simulink model "DBX_control_harness"  (R2015a)
settings: Solver=ode2  SolverMode=SingleTasking  StartTime=0.0  StopTime=inf  FixedStep=T_sim  RelTol=1e-3
values from neighbouring files (symbols this model uses):
  airport_alt = 587.5    [Run_DBX.m]
  latitude = 40.463650    (= 40.46365)    [Run_DBX.m]
  longitude = -3.554389    [Run_DBX.m]
  T_ctrl = 0.01    [Run_DBX.m]
  T_sim = 0.01    [Run_DBX.m]
undefined symbols (not defined in the file or in its folder): accel_sigmas, Alt_0, DBX_PWM, delta_a_L_0_servo, delta_a_R_0_servo, delta_rv_L_0_servo, delta_rv_R_0_servo, eta_1_0_servo, eta_2_0_servo, eta_3_0_servo, Euler_0, Euler_dot_sigmas, Euler_sigmas, g, GPS_pos_sig, Initial_Omegas, Newton, omgea_b_sigmas, qbar_sigma, quaternion_sigmas, Raphson, Roll_pich_sens, sigbuilder_block, Speed_sigmas, TAS_0, tau_1_0, tau_2_0, tau_3_0, Throtle_sens, Volt_noise, Yaw_sens
libraries: DBX_model x14, commnoisgen2 x9, simulink x3, powerlib_meascontrol x2, utility x1
(part 2 of 2)

== system DBX_control_harness/DBX FCS/PWM Interface out/PWM Interface out: Agosto prototipo ==
  PWM1 : Inport
  PWM2 : Inport  Port=2
  PWM3 : Inport  Port=3
  PWM4 : Inport  Port=4
  PWM5 : Inport  Port=5
  PWM6 : Inport  Port=6
  PWM7 : Inport  Port=7
  PWM8 : Inport  Port=8
  Constant : Constant  Value=1500
  Constant1 : Constant  Value=1100
  Mux : Mux  Inputs=3
  Mux1 : Mux  Inputs=7
  Motores : Outport
  Servos : Outport  Port=2
  wires:
  Mux/1 -> Motores/1
  Mux1/1 -> Servos/1
  PWM1/1 -> Mux/1
  PWM2/1 -> Mux/2
  PWM3/1 -> Mux1/1
  PWM4/1 -> Mux1/2
  PWM5/1 -> Mux1/4
  PWM6/1 -> Mux1/5
  PWM7/1 -> Mux1/6
  PWM8/1 -> Mux1/7
  Constant/1 -> Mux1/3
  Constant1/1 -> Mux/3

== system DBX_control_harness/DBX FCS/PWM Interface out/PWM Interface out: VTOL ==
  PWM1 : Inport
  PWM2 : Inport  Port=2
  PWM3 : Inport  Port=3
  PWM4 : Inport  Port=4
  PWM5 : Inport  Port=5
  PWM6 : Inport  Port=6
  PWM7 : Inport  Port=7
  PWM8 : Inport  Port=8
  Constant1 : Constant  Commented=on  Value=1100
  Constant2 : Constant  Value=1500
  Mux : Mux  Inputs=3
  Mux1 : Mux  Inputs=7
  Motores : Outport
  Servos : Outport  Port=2
  wires:
  Mux1/1 -> Servos/1
  Mux/1 -> Motores/1
  PWM1/1 -> Mux/1
  PWM2/1 -> Mux/2
  PWM3/1 -> Mux/3
  PWM4/1 -> Mux1/1
  PWM5/1 -> Mux1/2
  PWM6/1 -> Mux1/3
  PWM7/1 -> Mux1/4
  PWM8/1 -> Mux1/5
  Constant2/1 -> Mux1/7, Mux1/6

== system DBX_control_harness/DBX FCS/Simulink to px4 input/Flat Earth to LLA ==
  note: Flat Earth to LLA
  Xe : Inport
  altitude0 : Inport  Port=2
  Add : Sum
  Demux1 : Demux  Outputs=3
  Demux2 : Demux  Outputs=2
  Mux : Mux  Inputs=2
  Mux1 : Mux  Inputs=3
  Selector : Selector  InputPortWidth=3  Indices=3
  Unary Minus1 : UnaryMinus
  deg2rad : Gain  Gain=pi/180  SaturateOnIntegerOverflow=on  ParamDataTypeStr=Inherit: Same as input
  ne to lat/long : Subsystem
  latitude mu : Outport
  longitude l : Outport  Port=2
  altitude h : Outport  Port=3
  wires:
  Demux2/1 -> latitude mu/1  "latitude"
  Demux2/2 -> longitude l/1
  Xe/1 -> Demux1/1, Selector/1
  deg2rad/1 -> Demux2/1
  ne to lat/long/1(lat_deg) -> Mux/1
  ne to lat/long/2(long_deg) -> Mux/2
  Mux/1 -> deg2rad/1
  Selector/1 -> Unary Minus1/1
  Add/1 -> altitude h/1
  altitude0/1 -> Add/2
  Mux1/1 -> ne to lat/long/1(Xe)
  Demux1/1 -> Mux1/1
  Demux1/2 -> Mux1/2
  Demux1/3 -> Mux1/3
  Unary Minus1/1 -> Add/1

== system DBX_control_harness/FlightGear visualization/Flat Earth to LLA/ne to lat//long ==
  Xe : Inport
  Demux : Demux  Outputs=2
  "Latitude Between +/- 90 " : Subsystem  TreatAsAtomicUnit=on
  "LongLat_offset " : Subsystem  TreatAsAtomicUnit=on
  "Longitude Between +/-180 " : Subsystem  TreatAsAtomicUnit=on
  Sel1 : Selector  InputPortWidth=3  Indices=[1,2]
  Sum2 : Sum  Inputs=++|
  initial_latg : Constant  Value=latitude
  initial_pos : Constant  Value=[latitude,longitude]
  rad2deg : Gain  Gain=180/pi  SaturateOnIntegerOverflow=on  OutDataTypeStr=Inherit: Same as input  ParamDataTypeStr=Inherit: Same as input
  lat_deg : Outport
  long_deg : Outport  Port=2
  wires:
  Xe/1 -> Sel1/1
  Sum2/1 -> "Latitude Between +/- 90 "/1(mu l)
  "LongLat_offset "/1(DeltaLL_rad) -> rad2deg/1
  Sel1/1 -> "LongLat_offset "/1(XY)
  rad2deg/1 -> Sum2/2
  initial_pos/1 -> Sum2/1
  initial_latg/1 -> "LongLat_offset "/2(mu)
  "Latitude Between +/- 90 "/1("mu l ") -> "Longitude Between +/-180 "/1(mu l)
  "Longitude Between +/-180 "/1("mu l ") -> Demux/1
  Demux/1 -> lat_deg/1
  Demux/2 -> long_deg/1

== system DBX_control_harness/Pilot control /Logitec /Togle switch ==
  In1 : Inport
  Bias : Bias  Bias=-1
  Bistable : powerlib_meascontrol/Logic/Bistable  Qpriority=Reset  ic=0  Ts=-1
  Detect Increase : simulink/Logic and Bit Operations/Detect Increase  vinit=0.0  InputProcessing=Inherited  OutDataTypeStr=boolean
  Gain : Gain  Gain=2  ParamDataTypeStr=double
  Logical Operator : Logic  Operator=NOT  IconShape=distinctive  AllPortsSameDT=off  OutDataTypeStr=boolean
  Logical Operator1 : Logic  AllPortsSameDT=off  OutDataTypeStr=boolean
  Unit Delay : UnitDelay  SampleTime=-1
  Out1 : Outport
  wires:
  In1/1 -> Detect Increase/1
  Gain/1 -> Bias/1
  Detect Increase/1 -> Bistable/1, Logical Operator1/1
  Logical Operator1/1 -> Bistable/2
  Logical Operator/1 -> Logical Operator1/2
  Unit Delay/1 -> Logical Operator/1
  Bistable/2 -> Unit Delay/1
  Bistable/1 -> Gain/1
  Bias/1 -> Out1/1

== system DBX_control_harness/Pilot control /Logitec /Togle switch1 ==
  In1 : Inport
  Bias : Bias  Bias=-1
  Bistable : powerlib_meascontrol/Logic/Bistable  Qpriority=Reset  ic=0  Ts=-1
  Detect Increase : simulink/Logic and Bit Operations/Detect Increase  vinit=0.0  InputProcessing=Inherited  OutDataTypeStr=boolean
  Gain : Gain  Gain=2  ParamDataTypeStr=double
  Logical Operator : Logic  Operator=NOT  IconShape=distinctive  AllPortsSameDT=off  OutDataTypeStr=boolean
  Logical Operator1 : Logic  AllPortsSameDT=off  OutDataTypeStr=boolean
  Unit Delay : UnitDelay  SampleTime=-1
  Out1 : Outport
  wires:
  Bias/1 -> Out1/1
  Bistable/1 -> Gain/1
  Bistable/2 -> Unit Delay/1
  Unit Delay/1 -> Logical Operator/1
  Logical Operator/1 -> Logical Operator1/2
  Logical Operator1/1 -> Bistable/2
  Detect Increase/1 -> Logical Operator1/1, Bistable/1
  Gain/1 -> Bias/1
  In1/1 -> Detect Increase/1

== system DBX_control_harness/Pilot control /Signal generator/Signal Builder ==
  Demux : Demux  Tag=STV Demux  Outputs=2
  FromWs : FromWorkspace  Tag=STV FromWs  VariableName=tuvar  SampleTime=0
      SigBuilderData=|
      | common.afterFinalStr = 'Extrapolate'
      | common.sampleTime = 0
      | dataSet.timeRange = [0 20]
      | dataSet.name = 'Group 1'
      | sbobj.Groups.Name = 'Group 1'
      | sbobj.Groups.Signals(1).Name = 'Signal 1'
      | sbobj.Groups.Signals(1).XData = [0 4 4 6 6 20]
      | sbobj.Groups.Signals(1).YData = [0 0 0.49 0.49 0 0]
      | sbobj.Groups.Signals(2).Name = 'Signal 2'
      | sbobj.Groups.Signals(2).XData = [0 12 12 14 14 20]
      | sbobj.Groups.Signals(2).YData = [0 0 0.48 0.48 0 0]
      | sbobj.Groups.TimeRange = [0 20]
  Signal 1 : Outport  Tag=STV Outport
  Signal 2 : Outport  Tag=STV Outport  Port=2
  wires:
  Demux/1 -> Signal 1/1
  FromWs/1 -> Demux/1
  Demux/2 -> Signal 2/1

== system DBX_control_harness/Sensors and filtering. No noise/Sensors and filtering. NOISE/keep -pi//pi1 ==
  in (rad) : Inport
  Constant : Constant  Value=180
  Constant2 : Constant  Value=360
  Gain : Gain  Gain=360
  Math Function2 : Math  Operator=rem  SaturateOnIntegerOverflow=on
  Product : Product  Inputs=*/  RndMeth=Zero
  Rounding Function : Rounding  Operator=fix
  Sum2 : Sum  Inputs=|-+
  deg2rad1 : Gain  Gain=pi/180  SaturateOnIntegerOverflow=on  OutDataTypeStr=Inherit: Same as input  ParamDataTypeStr=Inherit: Same as input
  rad2deg : Gain  Gain=180/pi  SaturateOnIntegerOverflow=on  OutDataTypeStr=Inherit: Same as input  ParamDataTypeStr=Inherit: Same as input
  out (rad) : Outport
  wires:
  in (rad)/1 -> rad2deg/1
  Constant/1 -> Product/2
  Product/1 -> Rounding Function/1
  Rounding Function/1 -> Gain/1
  Gain/1 -> Sum2/1
  rad2deg/1 -> Math Function2/1
  Constant2/1 -> Math Function2/2
  Math Function2/1 -> Product/1, Sum2/2
  Sum2/1 -> deg2rad1/1
  deg2rad1/1 -> out (rad)/1

== system DBX_control_harness/Sensors and filtering. No noise/Sensors and filtering. No noise/keep -pi//pi1 ==
  in (rad) : Inport
  Constant : Constant  Value=180
  Constant2 : Constant  Value=360
  Gain : Gain  Gain=360
  Math Function2 : Math  Operator=rem  SaturateOnIntegerOverflow=on
  Product : Product  Inputs=*/  RndMeth=Zero
  Rounding Function : Rounding  Operator=fix
  Sum2 : Sum  Inputs=|-+
  deg2rad1 : Gain  Gain=pi/180  SaturateOnIntegerOverflow=on  OutDataTypeStr=Inherit: Same as input  ParamDataTypeStr=Inherit: Same as input
  rad2deg : Gain  Gain=180/pi  SaturateOnIntegerOverflow=on  OutDataTypeStr=Inherit: Same as input  ParamDataTypeStr=Inherit: Same as input
  out (rad) : Outport
  wires:
  deg2rad1/1 -> out (rad)/1
  Sum2/1 -> deg2rad1/1
  Math Function2/1 -> Sum2/2, Product/1
  Constant2/1 -> Math Function2/2
  rad2deg/1 -> Math Function2/1
  Gain/1 -> Sum2/1
  Rounding Function/1 -> Gain/1
  Product/1 -> Rounding Function/1
  Constant/1 -> Product/2
  in (rad)/1 -> rad2deg/1

== system DBX_control_harness/DBX FCS/Simulink to px4 input/Flat Earth to LLA/ne to lat//long ==
  Xe : Inport
  Demux : Demux  Outputs=2
  "Latitude Between +/- 90 " : Subsystem  TreatAsAtomicUnit=on
  "LongLat_offset " : Subsystem  TreatAsAtomicUnit=on
  "Longitude Between +/-180 " : Subsystem  TreatAsAtomicUnit=on
  Sel1 : Selector  InputPortWidth=3  Indices=[1,2]
  Sum2 : Sum  Inputs=++|
  initial_latg : Constant  Value=latitude
  initial_pos : Constant  Value=[latitude,longitude]
  rad2deg : Gain  Gain=180/pi  SaturateOnIntegerOverflow=on  OutDataTypeStr=Inherit: Same as input  ParamDataTypeStr=Inherit: Same as input
  lat_deg : Outport
  long_deg : Outport  Port=2
  wires:
  Xe/1 -> Sel1/1
  Sum2/1 -> "Latitude Between +/- 90 "/1(mu l)
  "LongLat_offset "/1(DeltaLL_rad) -> rad2deg/1
  Sel1/1 -> "LongLat_offset "/1(XY)
  rad2deg/1 -> Sum2/2
  initial_pos/1 -> Sum2/1
  initial_latg/1 -> "LongLat_offset "/2(mu)
  "Latitude Between +/- 90 "/1("mu l ") -> "Longitude Between +/-180 "/1(mu l)
  "Longitude Between +/-180 "/1("mu l ") -> Demux/1
  Demux/1 -> lat_deg/1
  Demux/2 -> long_deg/1

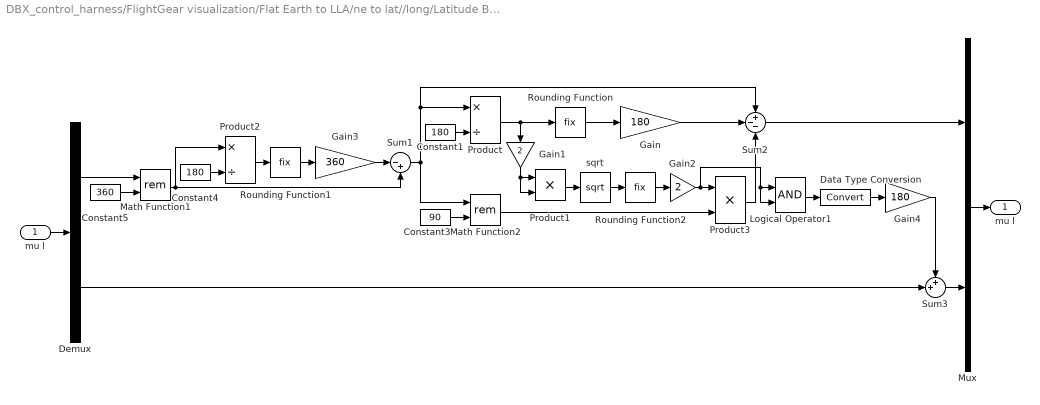
== system DBX_control_harness/FlightGear visualization/Flat Earth to LLA/ne to lat//long/Latitude Between +//- 90  ==
  mu l : Inport
  Constant1 : Constant  Value=180
  Constant3 : Constant  Value=90
  Constant4 : Constant  Value=180
  Constant5 : Constant  Value=360
  Data Type Conversion : DataTypeConversion
  Demux : Demux  Outputs=2
  Gain : Gain  Gain=180
  Gain1 : Gain  Gain=2
  Gain2 : Gain  Gain=2
  Gain3 : Gain  Gain=360
  Gain4 : Gain  Gain=180
  Logical Operator1 : Logic  AllPortsSameDT=off  OutDataTypeStr=boolean
  Math Function1 : Math  Operator=rem  SaturateOnIntegerOverflow=on
  Math Function2 : Math  Operator=rem  SaturateOnIntegerOverflow=on
  Mux : Mux  Inputs=2
  Product : Product  Inputs=*/  RndMeth=Zero
  Product1 : Product  RndMeth=Zero
  Product2 : Product  Inputs=*/  RndMeth=Zero
  Product3 : Product  RndMeth=Zero
  Rounding Function : Rounding  Operator=fix
  Rounding Function1 : Rounding  Operator=fix
  Rounding Function2 : Rounding  Operator=fix
  Sum1 : Sum  Inputs=|-+
  Sum2 : Sum  Inputs=+--
  Sum3 : Sum  Inputs=++|
  sqrt : Sqrt  AlgorithmType=Newton-Raphson  SaturateOnIntegerOverflow=on
  "mu l " : Outport
  wires:
  Sum3/1 -> Mux/2
  Demux/2 -> Sum3/2
  Demux/1 -> Math Function1/1
  mu l/1 -> Demux/1
  Mux/1 -> "mu l "/1
  Constant1/1 -> Product/2
  Product/1 -> Rounding Function/1, Gain1/1
  Rounding Function/1 -> Gain/1
  Gain/1 -> Sum2/2
  Sum2/1 -> Mux/1
  Constant3/1 -> Math Function2/2
  Math Function2/1 -> Product3/2
  Product3/1 -> Sum2/3
  Rounding Function2/1 -> Gain2/1
  Gain2/1 -> Product3/1, Logical Operator1/1, Logical Operator1/2
  Product1/1 -> sqrt/1
  sqrt/1 -> Rounding Function2/1
  Constant4/1 -> Product2/2
  Product2/1 -> Rounding Function1/1
  Rounding Function1/1 -> Gain3/1
  Gain3/1 -> Sum1/1
  Math Function1/1 -> Sum1/2, Product2/1
  Sum1/1 -> Math Function2/1, Product/1, Sum2/1
  Constant5/1 -> Math Function1/2
  Logical Operator1/1 -> Data Type Conversion/1
  Gain4/1 -> Sum3/1
  Data Type Conversion/1 -> Gain4/1
  Gain1/1 -> Product1/2, Product1/1

== system DBX_control_harness/FlightGear visualization/Flat Earth to LLA/ne to lat//long/LongLat_offset  ==
  XY : Inport
  mu : Inport  Port=2
  " " : Trigonometry
  "  " : Trigonometry  Operator=cos
  Demux : Demux  Outputs=2
  "Find Radian/Distance " : Subsystem  TreatAsAtomicUnit=on
  Mux : Mux  Inputs=2
  Sum : Sum  Inputs=|+-
  Sum1 : Sum  Inputs=|++
  deg2rad : Gain  Gain=pi/180  SaturateOnIntegerOverflow=on  OutDataTypeStr=Inherit: Same as input  ParamDataTypeStr=Inherit: Same as input
  rad lat : Product  RndMeth=Zero
  "rad long " : Product  RndMeth=Zero
  ref_pos : Constant  Value=0
  x*cos : Product  RndMeth=Zero
  x*sin : Product  RndMeth=Zero
  y*cos : Product  RndMeth=Zero
  y*sin : Product  RndMeth=Zero
  DeltaLL_rad : Outport
  wires:
  mu/1 -> "Find Radian/Distance "/1(mu)
  "Find Radian/Distance "/1(dNorth) -> rad lat/2
  "Find Radian/Distance "/2(dEast) -> "rad long "/1
  rad lat/1 -> Mux/1
  "rad long "/1 -> Mux/2
  Mux/1 -> DeltaLL_rad/1
  deg2rad/1 -> "  "/1, " "/1
  Demux/2 -> y*cos/1, y*sin/1
  Sum1/1 -> "rad long "/2
  y*cos/1 -> Sum1/2
  x*sin/1 -> Sum1/1
  Sum/1 -> rad lat/1
  y*sin/1 -> Sum/2
  " "/1 -> x*sin/2, y*sin/2
  x*cos/1 -> Sum/1
  "  "/1 -> y*cos/2, x*cos/2
  Demux/1 -> x*sin/1, x*cos/1
  XY/1 -> Demux/1
  ref_pos/1 -> deg2rad/1

== system DBX_control_harness/FlightGear visualization/Flat Earth to LLA/ne to lat//long/Longitude Between +//-180  ==
  mu l : Inport
  Constant : Constant  Value=180
  Constant2 : Constant  Value=360
  Demux1 : Demux  Outputs=2
  Gain : Gain  Gain=360
  Math Function2 : Math  Operator=rem  SaturateOnIntegerOverflow=on
  Mux1 : Mux  Inputs=2
  Product : Product  Inputs=*/  RndMeth=Zero
  Rounding Function : Rounding  Operator=fix
  Sum2 : Sum  Inputs=|-+
  "mu l " : Outport
  wires:
  Mux1/1 -> "mu l "/1
  Demux1/1 -> Mux1/1
  mu l/1 -> Demux1/1
  Constant/1 -> Product/2
  Product/1 -> Rounding Function/1
  Rounding Function/1 -> Gain/1
  Gain/1 -> Sum2/1
  Sum2/1 -> Mux1/2
  Demux1/2 -> Math Function2/1
  Constant2/1 -> Math Function2/2
  Math Function2/1 -> Product/1, Sum2/2

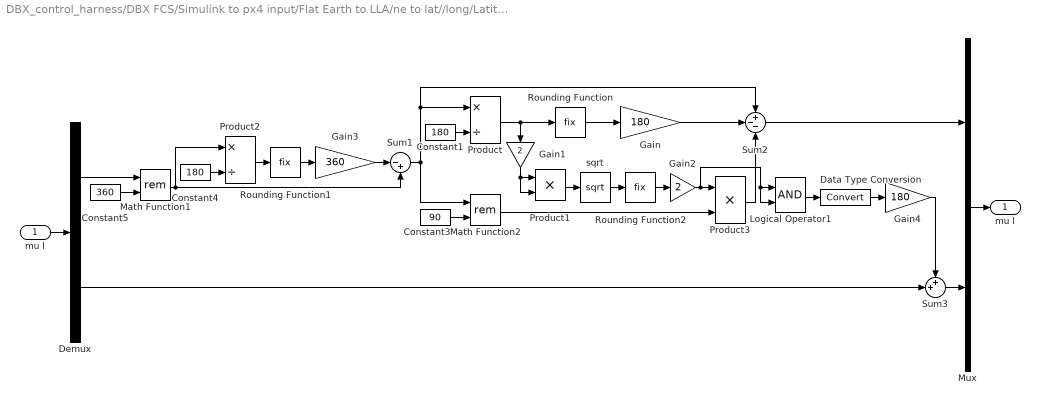
== system DBX_control_harness/DBX FCS/Simulink to px4 input/Flat Earth to LLA/ne to lat//long/Latitude Between +//- 90  ==
  mu l : Inport
  Constant1 : Constant  Value=180
  Constant3 : Constant  Value=90
  Constant4 : Constant  Value=180
  Constant5 : Constant  Value=360
  Data Type Conversion : DataTypeConversion
  Demux : Demux  Outputs=2
  Gain : Gain  Gain=180
  Gain1 : Gain  Gain=2
  Gain2 : Gain  Gain=2
  Gain3 : Gain  Gain=360
  Gain4 : Gain  Gain=180
  Logical Operator1 : Logic  AllPortsSameDT=off  OutDataTypeStr=boolean
  Math Function1 : Math  Operator=rem  SaturateOnIntegerOverflow=on
  Math Function2 : Math  Operator=rem  SaturateOnIntegerOverflow=on
  Mux : Mux  Inputs=2
  Product : Product  Inputs=*/  RndMeth=Zero
  Product1 : Product  RndMeth=Zero
  Product2 : Product  Inputs=*/  RndMeth=Zero
  Product3 : Product  RndMeth=Zero
  Rounding Function : Rounding  Operator=fix
  Rounding Function1 : Rounding  Operator=fix
  Rounding Function2 : Rounding  Operator=fix
  Sum1 : Sum  Inputs=|-+
  Sum2 : Sum  Inputs=+--
  Sum3 : Sum  Inputs=++|
  sqrt : Sqrt  AlgorithmType=Newton-Raphson  SaturateOnIntegerOverflow=on
  "mu l " : Outport
  wires:
  Sum3/1 -> Mux/2
  Demux/2 -> Sum3/2
  Demux/1 -> Math Function1/1
  mu l/1 -> Demux/1
  Mux/1 -> "mu l "/1
  Constant1/1 -> Product/2
  Product/1 -> Rounding Function/1, Gain1/1
  Rounding Function/1 -> Gain/1
  Gain/1 -> Sum2/2
  Sum2/1 -> Mux/1
  Constant3/1 -> Math Function2/2
  Math Function2/1 -> Product3/2
  Product3/1 -> Sum2/3
  Rounding Function2/1 -> Gain2/1
  Gain2/1 -> Product3/1, Logical Operator1/1, Logical Operator1/2
  Product1/1 -> sqrt/1
  sqrt/1 -> Rounding Function2/1
  Constant4/1 -> Product2/2
  Product2/1 -> Rounding Function1/1
  Rounding Function1/1 -> Gain3/1
  Gain3/1 -> Sum1/1
  Math Function1/1 -> Sum1/2, Product2/1
  Sum1/1 -> Math Function2/1, Product/1, Sum2/1
  Constant5/1 -> Math Function1/2
  Logical Operator1/1 -> Data Type Conversion/1
  Gain4/1 -> Sum3/1
  Data Type Conversion/1 -> Gain4/1
  Gain1/1 -> Product1/2, Product1/1

== system DBX_control_harness/DBX FCS/Simulink to px4 input/Flat Earth to LLA/ne to lat//long/LongLat_offset  ==
  XY : Inport
  mu : Inport  Port=2
  " " : Trigonometry
  "  " : Trigonometry  Operator=cos
  Demux : Demux  Outputs=2
  "Find Radian/Distance " : Subsystem  TreatAsAtomicUnit=on
  Mux : Mux  Inputs=2
  Sum : Sum  Inputs=|+-
  Sum1 : Sum  Inputs=|++
  deg2rad : Gain  Gain=pi/180  SaturateOnIntegerOverflow=on  OutDataTypeStr=Inherit: Same as input  ParamDataTypeStr=Inherit: Same as input
  rad lat : Product  RndMeth=Zero
  "rad long " : Product  RndMeth=Zero
  ref_pos : Constant  Value=0
  x*cos : Product  RndMeth=Zero
  x*sin : Product  RndMeth=Zero
  y*cos : Product  RndMeth=Zero
  y*sin : Product  RndMeth=Zero
  DeltaLL_rad : Outport
  wires:
  mu/1 -> "Find Radian/Distance "/1(mu)
  "Find Radian/Distance "/1(dNorth) -> rad lat/2
  "Find Radian/Distance "/2(dEast) -> "rad long "/1
  rad lat/1 -> Mux/1
  "rad long "/1 -> Mux/2
  Mux/1 -> DeltaLL_rad/1
  deg2rad/1 -> "  "/1, " "/1
  Demux/2 -> y*cos/1, y*sin/1
  Sum1/1 -> "rad long "/2
  y*cos/1 -> Sum1/2
  x*sin/1 -> Sum1/1
  Sum/1 -> rad lat/1
  y*sin/1 -> Sum/2
  " "/1 -> x*sin/2, y*sin/2
  x*cos/1 -> Sum/1
  "  "/1 -> y*cos/2, x*cos/2
  Demux/1 -> x*sin/1, x*cos/1
  XY/1 -> Demux/1
  ref_pos/1 -> deg2rad/1

== system DBX_control_harness/DBX FCS/Simulink to px4 input/Flat Earth to LLA/ne to lat//long/Longitude Between +//-180  ==
  mu l : Inport
  Constant : Constant  Value=180
  Constant2 : Constant  Value=360
  Demux1 : Demux  Outputs=2
  Gain : Gain  Gain=360
  Math Function2 : Math  Operator=rem  SaturateOnIntegerOverflow=on
  Mux1 : Mux  Inputs=2
  Product : Product  Inputs=*/  RndMeth=Zero
  Rounding Function : Rounding  Operator=fix
  Sum2 : Sum  Inputs=|-+
  "mu l " : Outport
  wires:
  Mux1/1 -> "mu l "/1
  Demux1/1 -> Mux1/1
  mu l/1 -> Demux1/1
  Constant/1 -> Product/2
  Product/1 -> Rounding Function/1
  Rounding Function/1 -> Gain/1
  Gain/1 -> Sum2/1
  Sum2/1 -> Mux1/2
  Demux1/2 -> Math Function2/1
  Constant2/1 -> Math Function2/2
  Math Function2/1 -> Product/1, Sum2/2

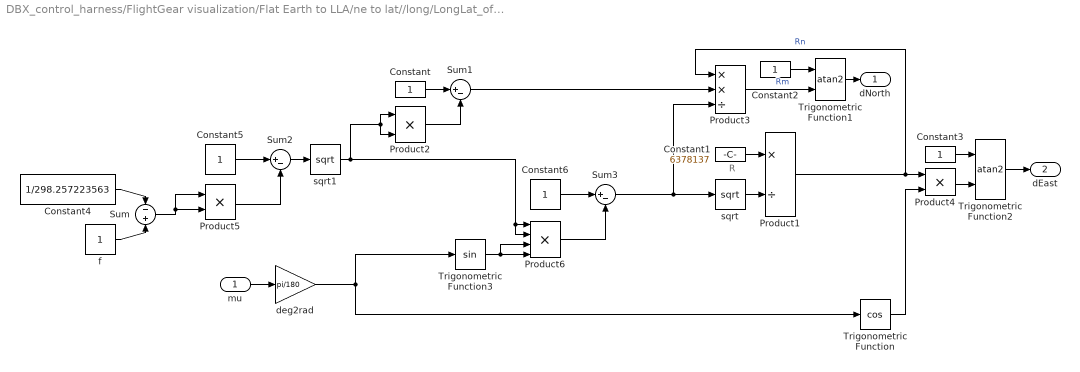
== system DBX_control_harness/FlightGear visualization/Flat Earth to LLA/ne to lat//long/LongLat_offset /Find Radian//Distance  ==
  note: R
  mu : Inport
  Constant{,2..3,5..6} (5 alike) : Constant
  Constant1 : Constant  Value=6378137
  Constant4 : Constant  Value=1/298.257223563
  Product1 : Product  Inputs=*/  RndMeth=Zero
  Product2 : Product  RndMeth=Zero
  Product3 : Product  Inputs=**/  RndMeth=Zero
  Product4 : Product  RndMeth=Zero
  Product5 : Product  RndMeth=Zero
  Product6 : Product  Inputs=4  RndMeth=Zero
  Sum : Sum  Inputs=-+
  Sum1 : Sum  Inputs=|+-
  Sum2 : Sum  Inputs=|+-
  Sum3 : Sum  Inputs=|+-
  Trigonometric Function : Trigonometry  Operator=cos
  Trigonometric Function1 : Trigonometry  Operator=atan2
  Trigonometric Function2 : Trigonometry  Operator=atan2
  Trigonometric Function3 : Trigonometry
  deg2rad : Gain  Gain=pi/180  SaturateOnIntegerOverflow=on  OutDataTypeStr=Inherit: Same as input  ParamDataTypeStr=Inherit: Same as input
  f : Constant
  sqrt : Sqrt  AlgorithmType=Newton-Raphson  SaturateOnIntegerOverflow=on
  sqrt1 : Sqrt  AlgorithmType=Newton-Raphson  SaturateOnIntegerOverflow=on
  dNorth : Outport
  dEast : Outport  Port=2
  wires:
  Trigonometric Function2/1 -> dEast/1
  Trigonometric Function1/1 -> dNorth/1
  Constant3/1 -> Trigonometric Function2/1
  Constant2/1 -> Trigonometric Function1/1
  Product4/1 -> Trigonometric Function2/2
  mu/1 -> deg2rad/1
  Trigonometric Function/1 -> Product4/2
  Product3/1 -> Trigonometric Function1/2  "Rm"
  Sum1/1 -> Product3/2
  Product1/1 -> Product4/1, Product3/1  "Rn"
  Constant/1 -> Sum1/1
  Product2/1 -> Sum1/2
  Constant1/1 -> Product1/1
  sqrt/1 -> Product1/2
  Sum3/1 -> Product3/3, sqrt/1
  f/1 -> Sum/2
  Constant4/1 -> Sum/1
  Sum/1 -> Product5/1, Product5/2
  Product5/1 -> Sum2/2
  Constant5/1 -> Sum2/1
  Sum2/1 -> sqrt1/1
  deg2rad/1 -> Trigonometric Function3/1, Trigonometric Function/1
  Trigonometric Function3/1 -> Product6/4, Product6/3
  sqrt1/1 -> Product6/1, Product6/2, Product2/2, Product2/1
  Product6/1 -> Sum3/2
  Constant6/1 -> Sum3/1

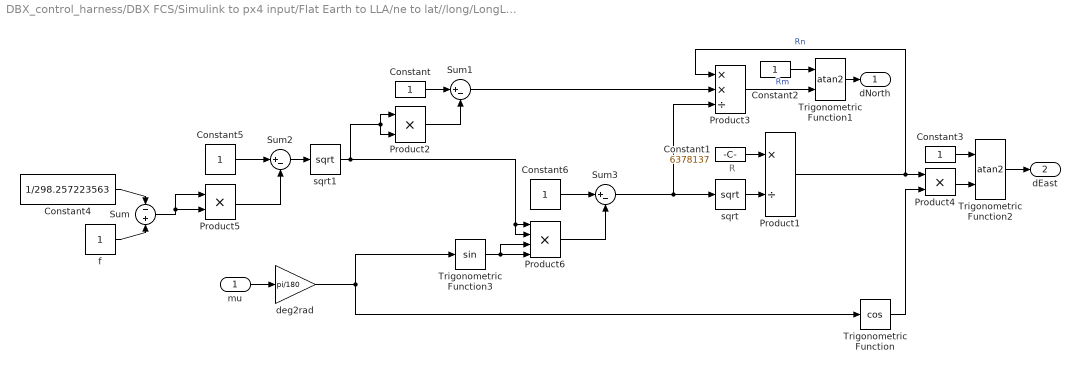
== system DBX_control_harness/DBX FCS/Simulink to px4 input/Flat Earth to LLA/ne to lat//long/LongLat_offset /Find Radian//Distance  ==
  note: R
  mu : Inport
  Constant{,2..3,5..6} (5 alike) : Constant
  Constant1 : Constant  Value=6378137
  Constant4 : Constant  Value=1/298.257223563
  Product1 : Product  Inputs=*/  RndMeth=Zero
  Product2 : Product  RndMeth=Zero
  Product3 : Product  Inputs=**/  RndMeth=Zero
  Product4 : Product  RndMeth=Zero
  Product5 : Product  RndMeth=Zero
  Product6 : Product  Inputs=4  RndMeth=Zero
  Sum : Sum  Inputs=-+
  Sum1 : Sum  Inputs=|+-
  Sum2 : Sum  Inputs=|+-
  Sum3 : Sum  Inputs=|+-
  Trigonometric Function : Trigonometry  Operator=cos
  Trigonometric Function1 : Trigonometry  Operator=atan2
  Trigonometric Function2 : Trigonometry  Operator=atan2
  Trigonometric Function3 : Trigonometry
  deg2rad : Gain  Gain=pi/180  SaturateOnIntegerOverflow=on  OutDataTypeStr=Inherit: Same as input  ParamDataTypeStr=Inherit: Same as input
  f : Constant
  sqrt : Sqrt  AlgorithmType=Newton-Raphson  SaturateOnIntegerOverflow=on
  sqrt1 : Sqrt  AlgorithmType=Newton-Raphson  SaturateOnIntegerOverflow=on
  dNorth : Outport
  dEast : Outport  Port=2
  wires:
  Trigonometric Function2/1 -> dEast/1
  Trigonometric Function1/1 -> dNorth/1
  Constant3/1 -> Trigonometric Function2/1
  Constant2/1 -> Trigonometric Function1/1
  Product4/1 -> Trigonometric Function2/2
  mu/1 -> deg2rad/1
  Trigonometric Function/1 -> Product4/2
  Product3/1 -> Trigonometric Function1/2  "Rm"
  Sum1/1 -> Product3/2
  Product1/1 -> Product4/1, Product3/1  "Rn"
  Constant/1 -> Sum1/1
  Product2/1 -> Sum1/2
  Constant1/1 -> Product1/1
  sqrt/1 -> Product1/2
  Sum3/1 -> Product3/3, sqrt/1
  f/1 -> Sum/2
  Constant4/1 -> Sum/1
  Sum/1 -> Product5/1, Product5/2
  Product5/1 -> Sum2/2
  Constant5/1 -> Sum2/1
  Sum2/1 -> sqrt1/1
  deg2rad/1 -> Trigonometric Function3/1, Trigonometric Function/1
  Trigonometric Function3/1 -> Product6/4, Product6/3
  sqrt1/1 -> Product6/1, Product6/2, Product2/2, Product2/1
  Product6/1 -> Sum3/2
  Constant6/1 -> Sum3/1

== matlab function DBX_control_harness/Pilot control /Logitec /Modo FCS ==
  data: s1 input; s2 input
function fcn(s1, s2)

eml.extrinsic('set_param','get_param','gcs');

if s1 > 0
    if s2 > 0
        set_param(get_param(get_param(gcs,'Parent'),'Parent'),'BackgroundColor','green');
    else
        set_param(get_param(get_param(gcs,'Parent'),'Parent'),'BackgroundColor','red');
    end
else
     set_param(get_param(get_param(gcs,'Parent'),'Parent'),'BackgroundColor','white');
end

== matlab function DBX_control_harness/Parameters estimation/MATLAB Function ==
  data: T_yaw output; yaw input
function T_yaw = Yaw_rotate(yaw)


T_yaw=[cos(yaw),    sin(yaw),   0;
        -sin(yaw),  cos(yaw),   0;
        0,      0,              1];
